simulink model "prova01"  (R2022b)
settings: Solver=VariableStepAuto  StartTime=0.0  StopTime=3600*9  RelTol=1e-3
values from neighbouring files (symbols this model uses):
  weatherSim =     [WeatherSim.mat]
settings Model: Creator=giaco  LastModifiedBy=giaco

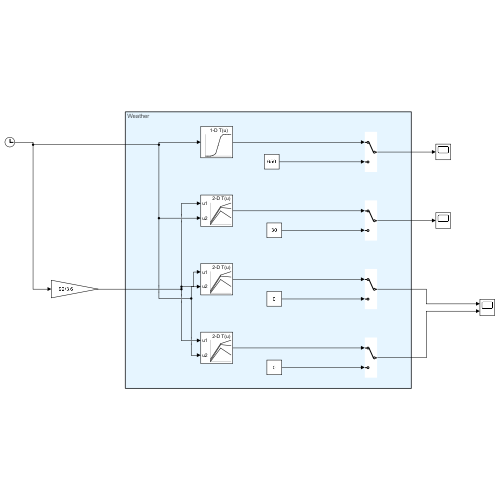
[thumbnail: Simulink's stored preview of the top-level diagram]
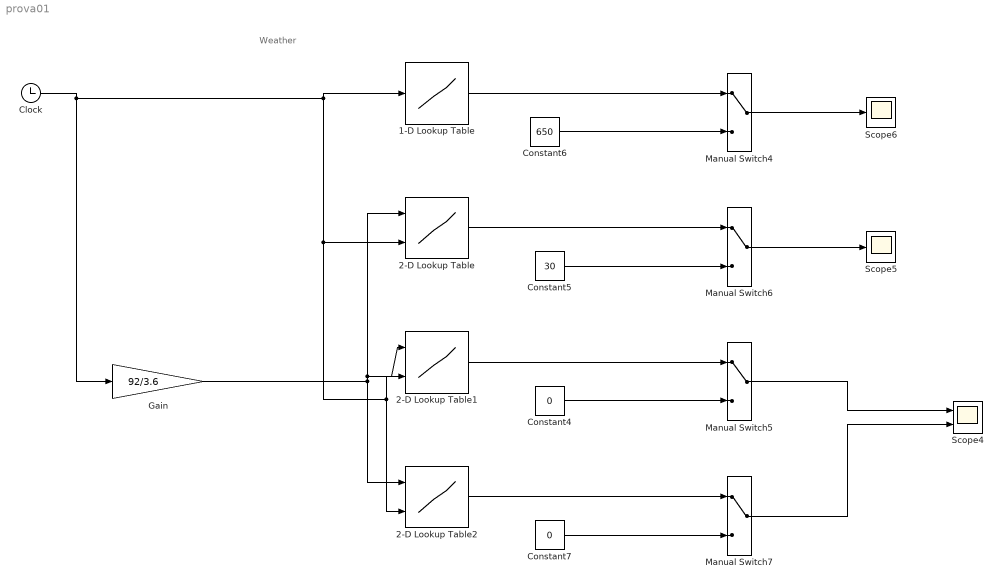
== system prova01 ==
  note: Weather
  1-D Lookup Table : Lookup_n-D  NumberOfTableDimensions=1  BreakpointsForDimension1=weatherSim.irradiance.timeSec  Table=weatherSim.irradiance.GtotalSec  InternalRulePriority=Speed  RndMeth=Simplest
  2-D Lookup Table : Lookup_n-D  BreakpointsForDimension1=weatherSim.temperature.dist  BreakpointsForDimension2=weatherSim.temperature.timeSec  Table=weatherSim.temperature.tempMean  InternalRulePriority=Speed  RndMeth=Simplest
      settings: InputPortMap=u0,u1
  2-D Lookup Table1 : Lookup_n-D  BreakpointsForDimension1=weatherSim.wind.dist  BreakpointsForDimension2=weatherSim.wind.timeSec  Table=weatherSim.wind.windMean  InternalRulePriority=Speed  RndMeth=Simplest
      settings: InputPortMap=u0,u1
  2-D Lookup Table2 : Lookup_n-D  BreakpointsForDimension1=weatherSim.wind.dist(1:end-1)  BreakpointsForDimension2=weatherSim.wind.timeSec  Table=weatherSim.wind.frontWind  InternalRulePriority=Speed  RndMeth=Simplest
      settings: InputPortMap=u0,u1
  Clock : Clock
  Constant4 : Constant  Value=0
  Constant5 : Constant  Value=30
  Constant6 : Constant  Value=650
  Constant7 : Constant  Value=0
  Gain : Gain  Gain=92/3.6
  Manual Switch{4..7} (4 alike) : ManualSwitch
  Scope4 : Scope  NumInputPorts=2
  Scope5 : Scope
  Scope6 : Scope
  wires:
  Constant6/1 -> Manual Switch4/2
  1-D Lookup Table/1 -> Manual Switch4/1
  2-D Lookup Table/1 -> Manual Switch6/1
  2-D Lookup Table1/1 -> Manual Switch5/1
  Constant4/1 -> Manual Switch5/2
  Constant7/1 -> Manual Switch7/2
  Constant5/1 -> Manual Switch6/2
  Manual Switch7/1 -> Scope4/2
  Manual Switch4/1 -> Scope6/1
  2-D Lookup Table2/1 -> Manual Switch7/1
  Gain/1 -> 2-D Lookup Table1/1, 2-D Lookup Table/1, 2-D Lookup Table2/1
  Clock/1 -> 1-D Lookup Table/1, 2-D Lookup Table/2, 2-D Lookup Table2/2, 2-D Lookup Table1/2, Gain/1
  Manual Switch5/1 -> Scope4/1
  Manual Switch6/1 -> Scope5/1
